simulink library "lib1"  (R2021a)
settings: Solver=VariableStepAuto  StartTime=0.0  StopTime=10.0  RelTol=1e-3
libraries: simulink x4, $bdroot x1
settings Model: Creator=yhd  LastModifiedBy=xbdz
settings SolverCC: AlgebraicLoopSolver=TrustRegion
settings DebuggingCC: SFMachineParentedDataDiag=warning
settings SFSimCC: CustomCodeUndefinedFunction=UseInterfaceOnly

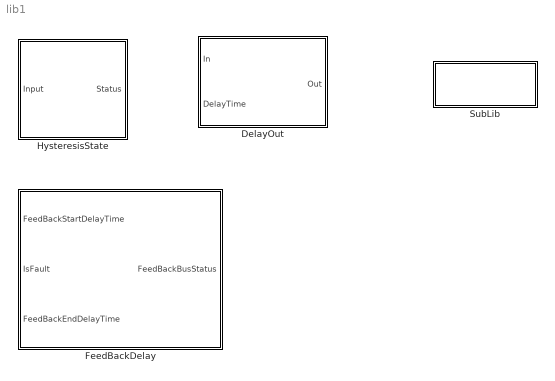
== system lib1 ==
  DelayOut : Subsystem  TreatAsAtomicUnit=on
      settings: RTWFcnNameOpts=Use subsystem name
  FeedBackDelay : Subsystem  TreatAsAtomicUnit=on
      settings: RTWFcnNameOpts=Use subsystem name
  HysteresisState : Stateflow chart  TreatAsAtomicUnit=on  mask{LowEntryTHR=1, LowExitTHR=2, HighEntryTHR=5, HighExitTHR=4, DelayCntTHR=2}
      mask prompts: LowEntryTHR "进入Low状态的阈值"; LowExitTHR "退出Low状态的阈值"; HighEntryTHR "进入High状态的阈值"; HighExitTHR "退出High状态的阈值"; DelayCntTHR "时间次数滞环阈值"
  SubLib : Subsystem
      settings: OpenFcn=sublib

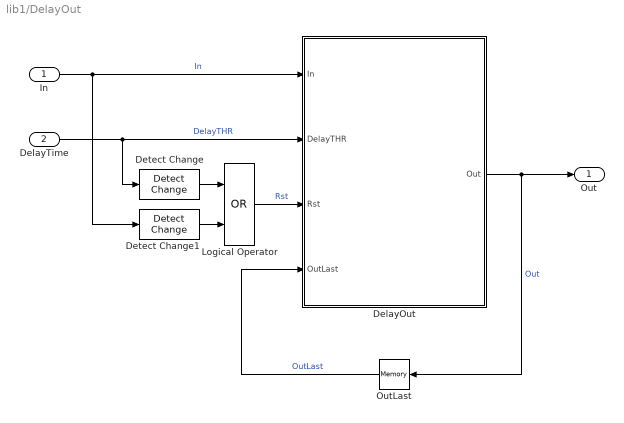
== system lib1/DelayOut ==
  In : Inport
  DelayTime : Inport  Port=2
  DelayOut : Stateflow chart  TreatAsAtomicUnit=on
  Detect Change : simulink/Logic and Bit Operations/Detect Change  vinit=0  OutDataTypeStr=boolean
  Detect Change1 : simulink/Logic and Bit Operations/Detect Change  vinit=0  OutDataTypeStr=boolean
  Logical Operator : Logic  Operator=OR  AllPortsSameDT=off  OutDataTypeStr=boolean
  OutLast : Memory  InheritSampleTime=on
  Out : Outport  VectorParamsAs1DForOutWhenUnconnected=off
  wires:
  In/1 -> Detect Change1/1, DelayOut/1(In)  "In"
  OutLast/1 -> DelayOut/4(OutLast)  "OutLast"
  Logical Operator/1 -> DelayOut/3(Rst)  "Rst"
  Detect Change1/1 -> Logical Operator/2
  Detect Change/1 -> Logical Operator/1
  DelayOut/1(Out) -> OutLast/1, Out/1  "Out"
  DelayTime/1 -> Detect Change/1, DelayOut/2(DelayTHR)  "DelayTHR"

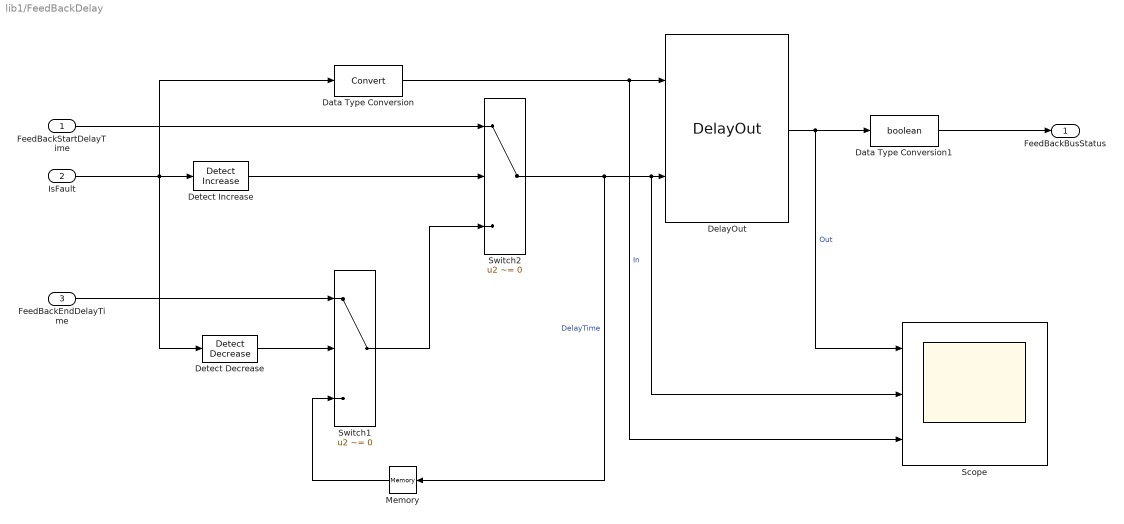
== system lib1/FeedBackDelay ==
  FeedBackStartDelayTime : Inport  OutDataTypeStr=uint16
  IsFault : Inport  Port=2  OutDataTypeStr=boolean
  FeedBackEndDelayTime : Inport  Port=3  OutDataTypeStr=uint16
  Data Type Conversion : DataTypeConversion
  Data Type Conversion1 : DataTypeConversion  OutDataTypeStr=boolean
  DelayOut : $bdroot/DelayOut  SystemSampleTime=-1  VariantActivationTime=update diagram  Latency=0  AutoFrameSizeCalculation=off
  Detect Decrease : simulink/Logic and Bit Operations/Detect Decrease  vinit=0.0  OutDataTypeStr=boolean
  Detect Increase : simulink/Logic and Bit Operations/Detect Increase  vinit=0.0  OutDataTypeStr=boolean
  Memory : Memory  InheritSampleTime=on
  Scope : Scope  NumInputPorts=3
  Switch1 : Switch  Criteria=u2 ~= 0
  Switch2 : Switch  Criteria=u2 ~= 0
  FeedBackBusStatus : Outport  VectorParamsAs1DForOutWhenUnconnected=off
  wires:
  Detect Decrease/1 -> Switch1/2
  Switch1/1 -> Switch2/3
  Detect Increase/1 -> Switch2/2
  IsFault/1 -> Data Type Conversion/1, Detect Decrease/1, Detect Increase/1
  Switch2/1 -> Memory/1, DelayOut/2, Scope/2  "DelayTime"
  Memory/1 -> Switch1/3
  DelayOut/1 -> Scope/1, Data Type Conversion1/1  "Out"
  Data Type Conversion/1 -> DelayOut/1, Scope/3  "In"
  FeedBackStartDelayTime/1 -> Switch2/1
  FeedBackEndDelayTime/1 -> Switch1/1
  Data Type Conversion1/1 -> FeedBackBusStatus/1

== system lib1/SubLib ==

== stateflow chart lib1/DelayOut/DelayOut ==
  state Delay
    Delay -> (junction 71) [order 1]
    (junction 71) -> (junction 72) [order 1] : [DelayCnt < DelayTHR]
        | {DelayCnt = DelayCnt + 1;
        | Out = OutLast;}
    (junction 71) -> (junction 73) [order 2]
    (junction 74) -> (junction 72)
    (junction 73) -> (junction 74) : {Out = In;}
  state Reset
    en:
    DelayCnt = 2;
    Out = OutLast;
    (junction 65) -> (junction 66) [order 1] : [DelayTHR == 0]
        | {Out = In;}
    Reset -> (junction 65) [order 1]
    (junction 65) -> (junction 66) [order 2]
  state DirectOut
    en:
    Out = In;
    du:
    Out = In;
  Reset -> Delay [order 2] : [Rst == false]
  (junction 56) -> Reset
  (junction 58) -> (junction 56) [order 2]
  Delay -> Reset [order 2] : [Rst == true]
  DirectOut -> Reset : [DelayTHR~= 0]
  Reset -> DirectOut [order 1] : [DelayTHR== 0]
  Delay -> (junction 81) [order 1] : [DelayTHR== 0]
  (default) -> (junction 58)
  (junction 58) -> DirectOut [order 1] : [DelayTHR== 0]
  (junction 81) -> DirectOut
  data: DelayCnt local uint16 =uint16(0); In input int16; Out output int16 =int16(0); DelayTHR input uint16; Rst input boolean; OutLast input int16

== stateflow chart lib1/HysteresisState ==
  state DefaultStatus
    en:
    IsInited=false;
    DefaultStatus -> (junction 78) [order 1]
    (junction 78) -> (junction 76) [order 1] : [Input>HighEntryTHR ]
        | {DefaultStatus = 1;}
    (junction 76) -> (junction 91) : {Status = DefaultStatus;
        | IsInited = true;}
    (junction 78) -> (junction 80) [order 2]
    (junction 82) -> (junction 76)
    (junction 80) -> (junction 82) [order 1] : [Input < LowEntryTHR]
        | {DefaultStatus = -1;}
    (junction 80) -> (junction 84) [order 2]
    (junction 86) -> (junction 82)
    (junction 84) -> (junction 86) : {DefaultStatus = 0;}
  state Normal
    entry:
    Status = 0;
    du:
    UpdateStateCnt(LowEntryTHR,HighEntryTHR);
  state Low
    entry:
    Status = -1;
    du:
    UpdateStateCnt(LowExitTHR+1,HighEntryTHR);
  note: Status:
      | 0:Normal
      | -1:Low
      | 1:High
  state High
    entry:
    Status = 1;
    du:
    UpdateStateCnt(LowEntryTHR,HighExitTHR-1);
  state UpdateStateCnt(lowTHR,highTHR) [function]
    (default) -> (junction 40)
    (junction 40) -> (junction 45) [order 2]
    (junction 45) -> (junction 49) [order 2]
    (junction 40) -> (junction 43) [order 1] : [Input < lowTHR]{
        | LowCnt = LowCnt + 1;
        | HighCnt = 0;
        | NormalCnt = 0;}
    (junction 45) -> (junction 47) [order 1] : [Input > highTHR]{
        | LowCnt = 0;
        | HighCnt = HighCnt + 1;
        | NormalCnt = 0;}
    (junction 49) -> (junction 51) : {LowCnt = 0;
        | HighCnt = 0;
        | NormalCnt = NormalCnt + 1;}
    (junction 47) -> (junction 43)
    (junction 51) -> (junction 47)
    (junction 43) -> (junction 53)
  (default) -> DefaultStatus
  DefaultStatus -> (junction 89) [order 1] : [IsInited == true]
  (junction 89) -> (junction 70) [order 3]
  (junction 89) -> (junction 67) [order 2] : [DefaultStatus == -1]
  (junction 70) -> (junction 72)
  (junction 89) -> Normal [order 1] : [DefaultStatus == 0]
  (junction 67) -> Low
  Normal -> Low [order 1] : [(Input < LowEntryTHR) ...
      | &&(LowCnt >= DelayCntTHR)]
  Low -> Normal [order 2] : [(Input > LowExitTHR) ...
      | &&(NormalCnt >= DelayCntTHR)]
  Low -> (junction 26) [order 1] : [(Input > HighEntryTHR) ...
      | &&(HighCnt >= DelayCntTHR)]
  (junction 29) -> Low
  Normal -> High [order 2] : [(Input > HighEntryTHR) ...
      | &&(HighCnt >= DelayCntTHR)]
  High -> Normal [order 2] : [(Input < HighExitTHR) ...
      | &&(NormalCnt >= DelayCntTHR)]
  (junction 26) -> High
  (junction 72) -> High
  High -> (junction 29) [order 1] : [(Input < LowEntryTHR) ...
      | &&(LowCnt >= DelayCntTHR)]
  data: lowTHR function_input int16; highTHR function_input int16; Input input int16; Status output int8 =int8(0); LowCnt local uint16 =uint16(0); HighCnt local uint16 =uint16(0); NormalCnt local uint16 =uint16(0); LowEntryTHR parameter int16; LowExitTHR parameter int16; HighEntryTHR parameter int16; HighExitTHR parameter int16; DelayCntTHR parameter uint16; DefaultStatus local int8; IsInited local boolean
